simulink model "control_architecture_gaussian_noise"  (R2024b)
settings: Solver=ode45  StartTime=0.0  StopTime=60  RelTol=1e-3
values from neighbouring files (symbols this model uses):
  DELTA = 0.001    [calculate_metrics_controlers.m]
  DERIVATIVE_PENALTY = 2.5    [calculate_metrics_controlers.m]
  EPSILON = 0.00005    (= 5e-05)    [calculate_metrics_controlers.m]
  INTEGRATIVE_PENALTY = 0.0003    [calculate_metrics_controlers.m]
  LAG = tmp.LAG    [optimize_input.m]
  MAX_ITER = 15    [calculate_metrics_controlers.m]
  Q = 1.6    [calculate_metrics_controlers.m]    (also in optimize_input.m = concatenated_vector((LAG*2+1)*5+1))
  ref = 50    [calculate_metrics_controlers.m]
  S = 0.0022    [calculate_metrics_controlers.m]
  X_max = concatenated_vector((LAG*2+1)*4+1:(LAG*2+1)*5)    [optimize_input.m]
  X_min = concatenated_vector((LAG*2+1)*3+1:(LAG*2+1)*4)    [optimize_input.m]
  Y_max = concatenated_vector((LAG*2+1)*12+1)    [optimize_input.m]
  Y_min = concatenated_vector((LAG*2+1)*11+1)    [optimize_input.m]
undefined symbols (not defined in the file or in its folder): control_init_vector_22
settings Model: Creator=gonzaloma  LastModifiedBy=gonzaloma

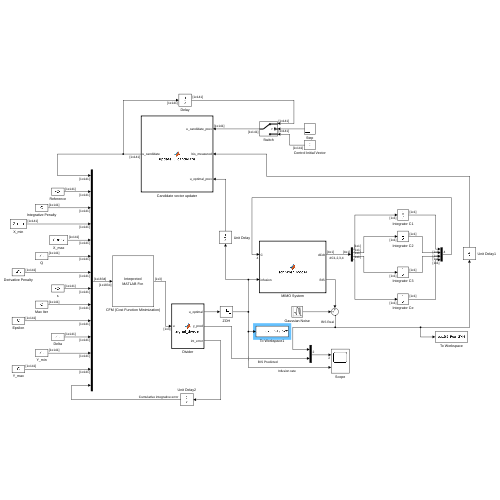
[thumbnail: Simulink's stored preview of the top-level diagram]
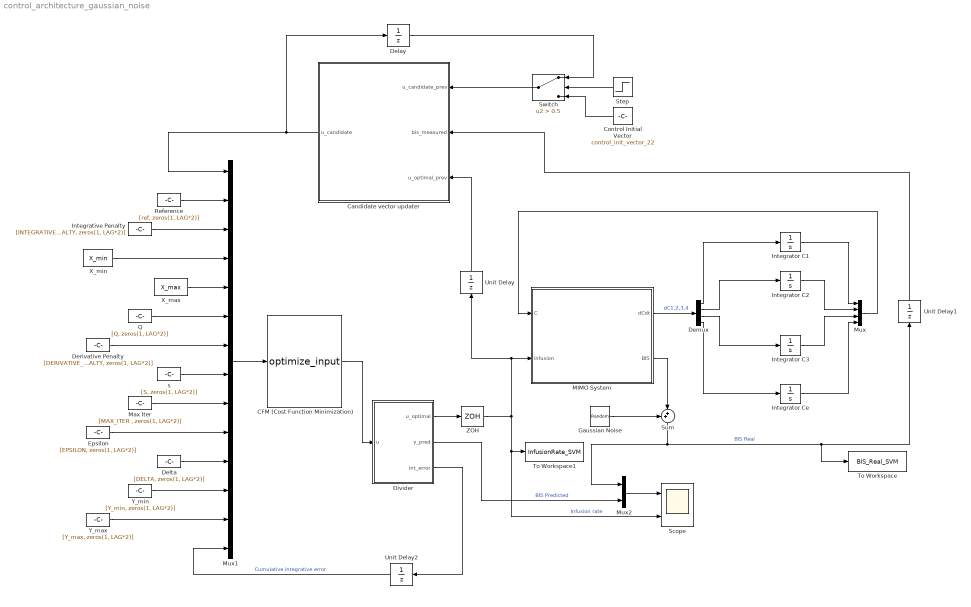
== system control_architecture_gaussian_noise ==
  CFM (Cost Function Minimization) : MATLABFcn  MATLABFcn=optimize_input  OutputDimensions=[1, 3]  Output1D=off
  Candidate vector updater : MATLAB Function  TreatAsAtomicUnit=on
  Control Initial Vector : Constant  Value=control_init_vector_22  VectorParams1D=off
  Delay : UnitDelay  SampleTime=-1  HasFrameUpgradeWarning=on
  Delta : Constant  Value=[DELTA, zeros(1, LAG*2)]  VectorParams1D=off
  Demux : Demux
  Derivative Penalty : Constant  Value=[DERIVATIVE_PENALTY, zeros(1, LAG*2)]  VectorParams1D=off
  Divider : MATLAB Function  TreatAsAtomicUnit=on
  Epsilon : Constant  Value=[EPSILON, zeros(1, LAG*2)]  VectorParams1D=off
  Gaussian Noise : RandomNumber  Seed=13  SampleTime=1/60
  Integrative Penalty : Constant  Value=[INTEGRATIVE_PENALTY, zeros(1, LAG*2)]  VectorParams1D=off
  Integrator C1 : Integrator  InitialCondition=1.7547
  Integrator C2 : Integrator  InitialCondition=0.17
  Integrator C3 : Integrator  InitialCondition=0.0759
  Integrator Ce : Integrator  InitialCondition=0.1658
  MIMO System : MATLAB Function  TreatAsAtomicUnit=on
  Max Iter : Constant  Value=[MAX_ITER , zeros(1, LAG*2)]  VectorParams1D=off
  Mux : Mux
  Mux1 : Mux  Inputs=14
  Mux2 : Mux  Inputs=2
  Q : Constant  Value=[Q, zeros(1, LAG*2)]  VectorParams1D=off
  Reference : Constant  Value=[ref, zeros(1, LAG*2)]  VectorParams1D=off
  Scope : Scope  NumInputPorts=2
  Step : Step  Time=0.001  SampleTime=0
  Sum : Sum  Inputs=++|
  Switch : Switch  Criteria=u2 > Threshold  Threshold=0.5  SaturateOnIntegerOverflow=off  InputSameDT=off
  To Workspace : ToWorkspace  VariableName=BIS_Real_SVM  SampleTime=-1
  To Workspace1 : ToWorkspace  VariableName=InfusionRate_SVM  SampleTime=-1
  Unit Delay : UnitDelay  InitialCondition=control_init_vector_22(LAG+1)  SampleTime=-1  HasFrameUpgradeWarning=on
  Unit Delay1 : UnitDelay  InitialCondition=control_init_vector_22(end)  SampleTime=-1  HasFrameUpgradeWarning=on
  Unit Delay2 : UnitDelay  SampleTime=-1  HasFrameUpgradeWarning=on
  X_max : Constant  Value=X_max  VectorParams1D=off
  X_min : Constant  Value=X_min  VectorParams1D=off
  Y_max : Constant  Value=[Y_max, zeros(1, LAG*2)]  VectorParams1D=off
  Y_min : Constant  Value=[Y_min, zeros(1, LAG*2)]  VectorParams1D=off
  ZOH : ZeroOrderHold  SampleTime=-1
  s : Constant  Value=[S, zeros(1, LAG*2)]  VectorParams1D=off
  wires:
  MIMO System/1(dCdt) -> Demux/1  "dC1,2,3,4"
  Demux/1 -> Integrator C1/1
  Demux/2 -> Integrator C2/1
  Demux/3 -> Integrator C3/1
  Demux/4 -> Integrator Ce/1
  Integrator C1/1 -> Mux/1
  Integrator C2/1 -> Mux/2
  Integrator C3/1 -> Mux/3
  Integrator Ce/1 -> Mux/4
  Mux/1 -> MIMO System/1(C)
  X_max/1 -> Mux1/5
  Candidate vector updater/1(u_candidate) -> Delay/1, Mux1/1
  Step/1 -> Switch/2
  Switch/1 -> Candidate vector updater/1(u_candidate_prev)
  Delay/1 -> Switch/1
  Control Initial Vector/1 -> Switch/3
  ZOH/1 -> To Workspace1/1, Scope/2, Unit Delay/1, MIMO System/2(infusion)  "Infusion rate"
  CFM (Cost Function Minimization)/1 -> Divider/1(u)
  Divider/1(u_optimal) -> ZOH/1
  Mux2/1 -> Scope/1
  Divider/2(y_pred) -> Mux2/2  "BIS Predicted"
  Mux1/1 -> CFM (Cost Function Minimization)/1
  Unit Delay/1 -> Candidate vector updater/3(u_optimal_prev)
  Divider/3(int_error) -> Unit Delay2/1
  Unit Delay2/1 -> Mux1/14  "Cumulative integrative error"
  Unit Delay1/1 -> Candidate vector updater/2(bis_measured)
  MIMO System/2(BIS) -> Sum/2
  Gaussian Noise/1 -> Sum/1
  Sum/1 -> Unit Delay1/1, To Workspace/1, Mux2/1  "BIS Real"
  Y_max/1 -> Mux1/13
  Epsilon/1 -> Mux1/10
  Derivative Penalty/1 -> Mux1/7
  Max Iter/1 -> Mux1/9
  Q/1 -> Mux1/6
  Y_min/1 -> Mux1/12
  X_min/1 -> Mux1/4
  Integrative Penalty/1 -> Mux1/3
  s/1 -> Mux1/8
  Delta/1 -> Mux1/11
  Reference/1 -> Mux1/2

== matlab function control_architecture_gaussian_noise/MIMO System ==
  settings: updateMethod=CONTINUOUS  sampleTime=1/60
  data: dCdt output size=[4, 1]; C input; infusion input; BIS output
function [dCdt, BIS] = schnider_model(C, infusion)
%#codegen

% Inputs:
%   t        - tiempo actual
%   C        - estado actual [C1; C2; C3; Ce]
%   infusion - tasa de infusión actual (u)
%   params   - estructura con parámetros

% Outputs:
%   dCdt - derivadas del estado
%   BIS  - salida (nivel BIS)

% Parametros
age = 28; % Age in years
weight = 60; % Weight in kg
height = 164; % Height in cm
gender = "M"; % Gender (M = Male; F = Female)

% Lean body mass calculation based on gender
if strcmp(gender, "M")
    LBM = (1.1 * weight) - 128 * (weight / height)^2; % Lean body mass (kg)
else
    LBM = (1.07 * weight) - 148 * (weight / height)^2; % Lean body mass (kg)
end

Ce50 = 4.93; % Effect site concentration for BIS 50 (mg/L)
gamma = 2.46; % Slope of the concentration-response curve

% Pharmacokinetic parameters of the Schnider model
V1 = 4.27; % Central compartment volume (L)
V2 = 18.9 - 0.391 * (age - 53); % Rapid peripheral compartment volume (L)
V3 = 238; % Slow peripheral compartment volume (L)

CL1 = 1.89 + ((weight - 77) * 0.0456) + ((LBM - 59) * (-0.0681)) + ((height - 177) * 0.0264); % Clearance of the central compartment (L/min)
CL2 = 1.29 - 0.024 * (age - 53); % Clearance between central and rapid peripheral compartment (L/min)
CL3 = 0.836; % Clearance between central and slow peripheral compartment (L/min)

% Transfer rate constants (calculated from clearances and volumes)
k10 = CL1 / V1;
k12 = CL2 / V1;
k13 = CL3 / V1;
k21 = CL2 / V2;
k31 = CL3 / V3;

% Pharmacodynamic (PD) effect-site parameters
ke0 = 0.456; % Rate constant for equilibrium between plasma and effect site (1/min)

% Additional parameters
BIS_base = 100; % Baseline BIS value (no drug effect)

% Dinámica PK (modelo de Schnider)
dCdt = zeros(4,1);
dCdt(1) = (infusion / V1) ...
          - k10*C(1) ...
          - k12*C(1) + k21*C(2) ...
          - k13*C(1) + k31*C(3);
      
dCdt(2) = k12*C(1) - k21*C(2);
dCdt(3) = k13*C(1) - k31*C(3);
dCdt(4) = ke0 * (C(1) - C(4)); % Sitio de efecto (Ce)

% Salida BIS
BIS = BIS_base * (Ce50^gamma) / (Ce50^gamma + C(4)^gamma);

== matlab function control_architecture_gaussian_noise/Candidate vector updater ==
  settings: updateMethod=DISCRETE  sampleTime=1/60
  data: u_candidate_prev input; u_candidate output; bis_measured input; u_optimal_prev input; LAG parameter
function u_candidate = update_u_candidate(u_candidate_prev, bis_measured, u_optimal_prev, LAG)   
    u_candidate = zeros(1, LAG*2+1);
    % Actualizar las entradas (shift left)
    u_candidate(1:LAG) = u_candidate_prev(2:LAG+1);
    
    % Colocar el último u aplicado en la posición correspondiente
    u_candidate(LAG+1) = u_optimal_prev;
    
    % Actualizar las salidas (shift left)
    u_candidate(LAG+2:end-1) = u_candidate_prev(LAG+3:end);
    
    % Insertar el BIS actual medido al final
    u_candidate(end) = bis_measured;
end

== matlab function control_architecture_gaussian_noise/Divider ==
  settings: updateMethod=DISCRETE  sampleTime=1/60
  data: u input; u_optimal output; y_pred output; int_error output
function [u_optimal, y_pred, int_error] = signal_divider(u)
   u_optimal = u(1);
   y_pred = u(2);
   int_error = u(3);
end
